simulink model "hot_water_storage_tank_simplified"  (R2017a)
settings: Solver=VariableStepAuto  StartTime=0.0  StopTime=50000  RelTol=1e-3
settings Model: Creator=info  LastModifiedBy=info

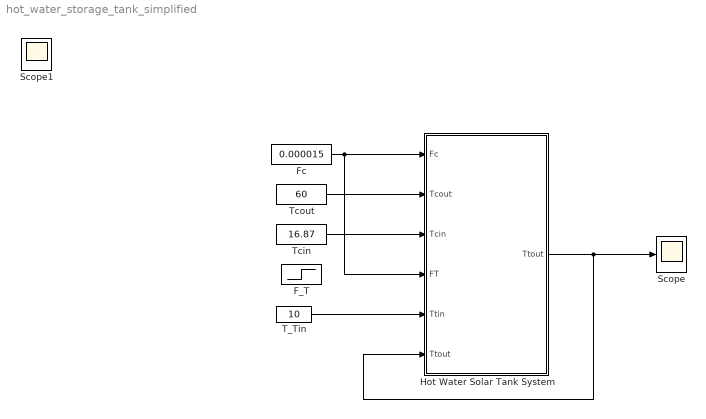
== system hot_water_storage_tank_simplified ==
  "F_T " : Step  Time=5  After=0.000015  SampleTime=0
  "Fc " : Constant  Value=0.000015
  Hot Water Solar Tank System : Subsystem
      mask Display: image('storage_tank.PNG');
  Scope : Scope
  T_Tin : Constant  Value=10
  Tcin : Constant  Value=16.87
  Tcout : Constant  Value=60
  Scope1 : Scope
  wires:
  Tcout/1 -> Hot Water Solar Tank System/2("Tcout ")
  T_Tin/1 -> Hot Water Solar Tank System/5("Ttin ")
  Hot Water Solar Tank System/1("Ttout ") -> Hot Water Solar Tank System/6(Ttout), Scope/1
  "Fc "/1 -> Hot Water Solar Tank System/4("FT "), Hot Water Solar Tank System/1("Fc ")
  Tcin/1 -> Hot Water Solar Tank System/3(Tcin)

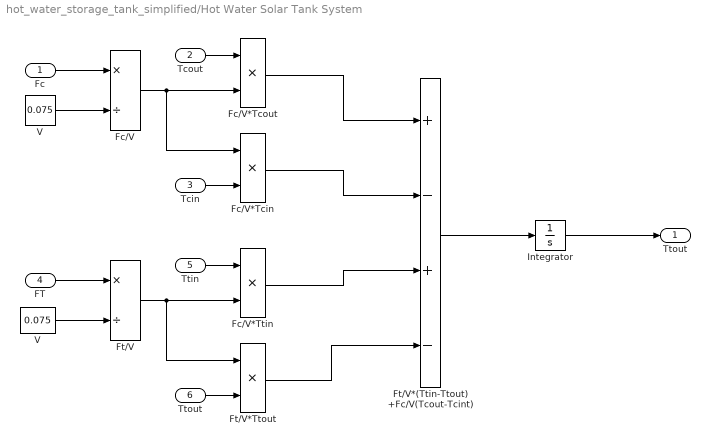
== system hot_water_storage_tank_simplified/Hot Water Solar Tank System ==
  "Fc " : Inport
  "Tcout " : Inport  Port=2
  Tcin : Inport  Port=3
  "FT " : Inport  Port=4
  "Ttin " : Inport  Port=5
  Ttout : Inport  Port=6
  Fc/V : Product  Inputs=*/
  Fc/V*Tcin : Product  Inputs=**
  Fc/V*Tcout : Product  Inputs=**
  Fc/V*Ttin : Product  Inputs=**
  Ft/V : Product  Inputs=*/
  Ft/V*(Ttin-Ttout) +Fc/V(Tcout-Tcint) : Sum  Inputs=+-+-
  Ft/V*Ttout : Product  Inputs=**
  Integrator : Integrator  InitialCondition=30
  V : Constant  Value=0.075
  "V " : Constant  Value=0.075
  "Ttout " : Outport
  wires:
  "Fc "/1 -> Fc/V/1
  Fc/V/1 -> Fc/V*Tcin/1, Fc/V*Tcout/2
  Integrator/1 -> "Ttout "/1
  "Tcout "/1 -> Fc/V*Tcout/1
  Fc/V*Tcout/1 -> Ft/V*(Ttin-Ttout) +Fc/V(Tcout-Tcint)/1
  Ft/V*(Ttin-Ttout) +Fc/V(Tcout-Tcint)/1 -> Integrator/1
  V/1 -> Fc/V/2
  Tcin/1 -> Fc/V*Tcin/2
  Ttout/1 -> Ft/V*Ttout/2
  "V "/1 -> Ft/V/2
  Fc/V*Ttin/1 -> Ft/V*(Ttin-Ttout) +Fc/V(Tcout-Tcint)/3
  "Ttin "/1 -> Fc/V*Ttin/1
  Ft/V/1 -> Fc/V*Ttin/2, Ft/V*Ttout/1
  "FT "/1 -> Ft/V/1
  Fc/V*Tcin/1 -> Ft/V*(Ttin-Ttout) +Fc/V(Tcout-Tcint)/2
  Ft/V*Ttout/1 -> Ft/V*(Ttin-Ttout) +Fc/V(Tcout-Tcint)/4
